simulink model "CM680A_HwTq2Meas"  (R2013b)
settings: Solver=FixedStepDiscrete  SolverMode=SingleTasking  StartTime=0.0  StopTime=1  FixedStep=0.002  RelTol=1e-3
values from neighbouring files (symbols this model uses):
  ELECGLBPRM_HWTQOFFS_HWNWTMTR_F32 = DataDict.Constant    [CM680A_HwTq2Meas_DataDict.m]
  ELECGLBPRM_HWTQSATNLOWRLIM_HWNWTMTR_F32 = DataDict.Constant    [CM680A_HwTq2Meas_DataDict.m]
  ELECGLBPRM_HWTQSATNUPPRLIM_HWNWTMTR_F32 = DataDict.Constant    [CM680A_HwTq2Meas_DataDict.m]
  ELECGLBPRM_HWTQSCA_ULS_F32 = DataDict.Constant    [CM680A_HwTq2Meas_DataDict.m]
  ELECGLBPRM_NOFLT_CNT_U08 = DataDict.Constant    [CM680A_HwTq2Meas_DataDict.m]
  ELECGLBPRM_OFFSTRIMNOTPRFM_CNT_U08 = DataDict.Constant    [CM680A_HwTq2Meas_DataDict.m]
  ELECGLBPRM_PRTCLFLT_CNT_U08 = DataDict.Constant    [CM680A_HwTq2Meas_DataDict.m]
  ELECGLBPRM_SNSRINTFLT_CNT_U08 = DataDict.Constant    [CM680A_HwTq2Meas_DataDict.m]
  FLTINJ_HWTQ2MEAS_HWTQ2 = DataDict.Constant    [CM680A_HwTq2Meas_DataDict.m]
  GearIdn1 = DataDict.OpSignal    [CM680A_HwTq2Meas_DataDict.m]
  HwTq2MeasHwTq2PrtclFltFailStep = DataDict.Calibration    [CM680A_HwTq2Meas_DataDict.m]
  HwTq2MeasHwTq2PrtclFltPassStep = DataDict.Calibration    [CM680A_HwTq2Meas_DataDict.m]
undefined symbols (not defined in the file or in its folder): NtcNr1, NtcSts1, sigbuilder_block, SigQlfr1
libraries: simulink x22, NxtrNvM x3
(part 2 of 3)

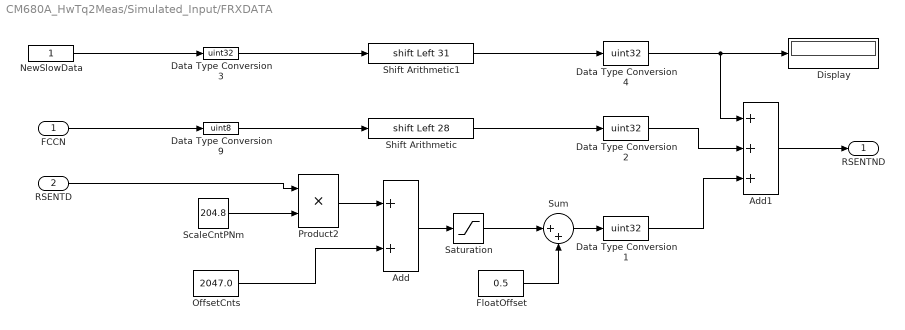
== system CM680A_HwTq2Meas/Simulated_Input/FRXDATA ==
  FCCN : Inport
  RSENTD : Inport  Port=2
  Add : Sum
  Add1 : Sum  Inputs=+++
  Data Type Conversion{1..4} (4 alike) : DataTypeConversion  OutDataTypeStr=uint32
  Data Type Conversion9 : DataTypeConversion  OutDataTypeStr=uint8
  Display : Display
  FloatOffset : Constant  Value=0.5
  NewSlowData : Constant
  OffsetCnts : Constant  Value=2047.0
  Product2 : Product
  Saturation : Saturate  UpperLimit=4095.0  LowerLimit=0.0
  ScaleCntPNm : Constant  Value=204.8
  Shift Arithmetic : ArithShift  BitShiftNumber=28  BitShiftDirection=Left
  Shift Arithmetic1 : ArithShift  BitShiftNumber=31  BitShiftDirection=Left
  Sum : Sum  Inputs=|++
  RSENTND : Outport
  wires:
  Data Type Conversion4/1 -> Add1/1, Display/1
  Shift Arithmetic1/1 -> Data Type Conversion4/1
  Data Type Conversion3/1 -> Shift Arithmetic1/1
  NewSlowData/1 -> Data Type Conversion3/1
  Data Type Conversion2/1 -> Add1/2
  Shift Arithmetic/1 -> Data Type Conversion2/1
  Add1/1 -> RSENTND/1
  Data Type Conversion1/1 -> Add1/3
  Data Type Conversion9/1 -> Shift Arithmetic/1
  FCCN/1 -> Data Type Conversion9/1
  Sum/1 -> Data Type Conversion1/1
  FloatOffset/1 -> Sum/2
  Saturation/1 -> Sum/1
  Add/1 -> Saturation/1
  OffsetCnts/1 -> Add/2
  Product2/1 -> Add/1
  ScaleCntPNm/1 -> Product2/2
  RSENTD/1 -> Product2/1

== system CM680A_HwTq2Meas/Simulated_Input/FRXDATA1 ==
  Snsr0CS : Inport
  Snsr0FRS : Inport  Port=2
  Add1 : Sum
  Data Type Conversion1 : DataTypeConversion  OutDataTypeStr=uint32
  Data Type Conversion9 : DataTypeConversion  OutDataTypeStr=uint32
  Shift Arithmetic2 : ArithShift  BitShiftNumber=1  BitShiftDirection=Left
  RSENTCS : Outport
  wires:
  Shift Arithmetic2/1 -> Add1/1
  Data Type Conversion9/1 -> Shift Arithmetic2/1
  Data Type Conversion1/1 -> Add1/2
  Snsr0FRS/1 -> Data Type Conversion1/1
  Add1/1 -> RSENTCS/1
  Snsr0CS/1 -> Data Type Conversion9/1

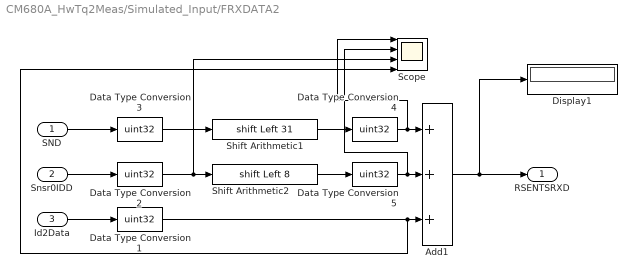
== system CM680A_HwTq2Meas/Simulated_Input/FRXDATA2 ==
  SND : Inport
  Snsr0IDD : Inport  Port=2
  Id2Data : Inport  Port=3
  Add1 : Sum  Inputs=+++
  Data Type Conversion{1..5} (5 alike) : DataTypeConversion  OutDataTypeStr=uint32
  Display1 : Display
  Scope : Scope  NumInputPorts=4
      settings: YMin=0~0~0~2  YMax=2.25e+09~1100~4~2
  Shift Arithmetic1 : ArithShift  BitShiftNumber=31  BitShiftDirection=Left
  Shift Arithmetic2 : ArithShift  BitShiftNumber=8  BitShiftDirection=Left
  RSENTSRXD : Outport
  wires:
  Id2Data/1 -> Data Type Conversion1/1
  Snsr0IDD/1 -> Data Type Conversion2/1
  Add1/1 -> RSENTSRXD/1, Display1/1
  SND/1 -> Data Type Conversion3/1
  Data Type Conversion3/1 -> Shift Arithmetic1/1
  Shift Arithmetic1/1 -> Data Type Conversion4/1
  Data Type Conversion4/1 -> Scope/1, Add1/1
  Data Type Conversion2/1 -> Scope/3, Shift Arithmetic2/1
  Data Type Conversion1/1 -> Scope/4, Add1/3
  Shift Arithmetic2/1 -> Data Type Conversion5/1
  Data Type Conversion5/1 -> Scope/2, Add1/2

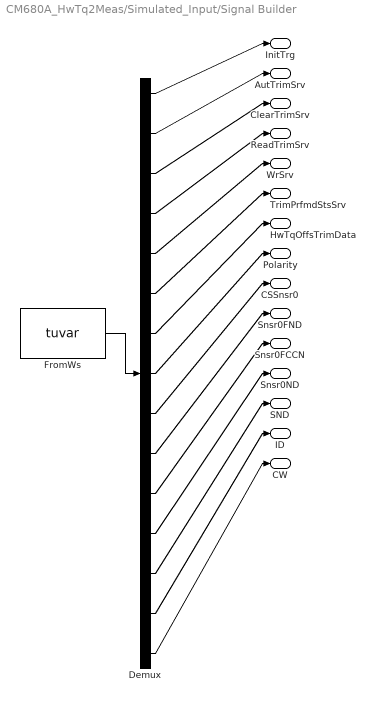
== system CM680A_HwTq2Meas/Simulated_Input/Signal Builder ==
  Demux : Demux  Tag=STV Demux  Outputs=15
  FromWs : FromWorkspace  Tag=STV FromWs  VariableName=tuvar  SampleTime=0  OutputAfterFinalValue=Holding final value
      SigBuilderData=|
      | common.afterFinalStr = 'Hold final value'
      | common.sampleTime = '0'
      | dataSet(1).timeRange = [0 20]
      | dataSet(1).name = 'IdealSignal'
      | dataSet(2).timeRange = [0 20]
      | dataSet(2).name = 'Faults'
      | dataSet(3).timeRange = [0 20]
      | dataSet(3).name = 'Service'
      | sbobj.Groups(1).Name = 'IdealSignal'
      | sbobj.Groups(1).Signals(1).Name = 'InitTrg'
      | sbobj.Groups(1).Signals(1).XData = [0 0.02 0.02 0.06 0.06 20]
      | sbobj.Groups(1).Signals(1).YData = [0 0 1 1 0 0]
      | sbobj.Groups(1).Signals(2).Name = 'AutTrimSrv'
      | sbobj.Groups(1).Signals(2).XData = [0 20]
      | sbobj.Groups(1).Signals(2).YData = [0 0]
      | sbobj.Groups(1).Signals(3).Name = 'ClearTrimSrv'
      | sbobj.Groups(1).Signals(3).XData = [0 20]
      | sbobj.Groups(1).Signals(3).YData = [0 0]
      | sbobj.Groups(1).Signals(4).Name = 'ReadTrimSrv'
      | sbobj.Groups(1).Signals(4).XData = [0 20]
      | sbobj.Groups(1).Signals(4).YData = [0 0]
      | sbobj.Groups(1).Signals(5).Name = 'WrSrv'
      | sbobj.Groups(1).Signals(5).XData = [0 0.04 0.04 0.08 0.08 20]
      | sbobj.Groups(1).Signals(5).YData = [0 0 1 1 0 0]
      | sbobj.Groups(1).Signals(6).Name = 'TrimPrfmdStsSrv'
      | sbobj.Groups(1).Signals(6).XData = [0 20]
      | sbobj.Groups(1).Signals(6).YData = [0 0]
      | sbobj.Groups(1).Signals(7).Name = 'HwTqOffsTrimData'
      | sbobj.Groups(1).Signals(7).XData = [0 20]
      | sbobj.Groups(1).Signals(7).YData = [0 0]
      | sbobj.Groups(1).Signals(8).Name = 'Polarity'
      | sbobj.Groups(1).Signals(8).XData = [0 20]
      | sbobj.Groups(1).Signals(8).YData = [1 1]
      | sbobj.Groups(1).Signals(9).Name = 'CSSnsr0'
      | sbobj.Groups(1).Signals(9).XData = [0 20]
      | sbobj.Groups(1).Signals(9).YData = [0 0]
      | sbobj.Groups(1).Signals(10).Name = 'Snsr0FND'
      | sbobj.Groups(1).Signals(10).XData = [0 20]
      | sbobj.Groups(1).Signals(10).YData = [1 1]
      | sbobj.Groups(1).Signals(11).Name = 'Snsr0FCCN'
      | sbobj.Groups(1).Signals(11).XData = [0 20]
      | sbobj.Groups(1).Signals(11).YData = [0 0]
      | sbobj.Groups(1).Signals(12).Name = 'Snsr0ND'
      | sbobj.Groups(1).Signals(12).XData = [0 2 2 4 4 6 6 8 8 10 10 12 12 14 14 16 16 18 18 20]
      | sbobj.Groups(1).Signals(12).YData = [-10 10 -10 10 -10 10 -10 10 -10 10 -10 10 -10 10 -10 10 -10 10 -10 10]
      | sbobj.Groups(1).Signals(13).Name = 'SND'
      | sbobj.Groups(1).Signals(13).XData = [0 0.1 0.1 0.2 0.2 0.3 0.3 0.4 0.4 0.5 0.5 0.6 0.6 0.7 0.7 0.8 0.8 0.9 0.9 1 1 1.1 1.1 1.2 1.2 1.3 1.3 1.4 1.4 1.5 1.5 1.6 1.6 1.7 1.7 1.8 1.8 1.9 1.9 2 2 2.1 2.1 2.2 2.2 2.3 2.3 2.4 2.4 2.5 2.5 2.6 2.6 2.7 2.7 2.8 2.8 2.9 2.9 3 3 3.1 3.1 3.2 3.2 3.3 3.3 3.4 3.4 3.5 3.5 3.6 3.6 3.7 3.7 3.8 3.8 3.9 3.9 4 4 4.1 4.1 4.2 4.2 4.3 4.3 4.4 4.4 4.5 4.5 4.6 4.6 4.7 4.7 4.8 4.8 4.9 4.9 5 5 5.1 5.1 5.2 5.2 5.3 5.3 5.4 5.4 5.5 5.5 5.6 5.6 5.7 5.7 5.8 5.8 5.9 5.9 6 6 6.1 6.1 6.2 6.2 6.3 6.3 6.4 6.4 6.5 6.5 6.6 6.6 6.7 6.7 6.8 6.8 6.9 6.9 7 7 7.1 7.1 7.2 7.2 7.3 7.3 7.4 7.4 7.5 7.5 7.6 7.6 7.7 7.7 7.8 7.8 7.9 7.9 8 8 8.1 8.1 8.2 8.2 8.3 8.3 8.4 8.4 8.5 8.5 8.6 8.6 8.7 8.7 8.8 8.8 8.9 8.9 9 9 9.1 9.1 9.2 9.2 9.3 9.3 9.4 9.4 9.5 9.5 9.6 9.6 9.7 9.7 9.8 9.8 9.9 9.9 10 10 10.1 10.1 10.2 10.2 10.3 10.3 10.4 10.4 10.5 10.5 10.6 10.6 10.7 10.7 10.8 10.8 10.9 10.9 11 11 11.1 11.1 11.2 11.2 11.3 11.3 11.4 11.4 11.5 11.5 11.6 11.6 11.7 11.7 11.8 11.8 11.9 11.9 12 12 12.1 12.1 12.2 12.2 12.3 12.3 12.4 12.4 12.5 12.5 12.6 12.6 12.7 12.7 12.8 12.8 12.9 12.9 13 13 13.1 13.1 13.2 13.2 13.3 13.3 13.4 13.4 13.5 13.5 13.6 13.6 13.7 13.7 13.8 13.8 13.9 13.9 14 14 14.1 14.1 14.2 14.2 14.3 14.3 14.4 14.4 14.5 14.5 14.6 14.6 14.7 14.7 14.8 14.8 14.9 14.9 15 15 15.1 15.1 15.2 15.2 15.3 15.3 15.4 15.4 15.5 15.5 15.6 15.6 15.7 15.7 15.8 15.8 15.9 15.9 16 16 16.1 16.1 16.2 16.2 16.3 16.3 16.4 16.4 16.5 16.5 16.6 16.6 16.7 16.7 16.8 16.8 16.9 16.9 17 17 17.1 17.1 17.2 17.2 17.3 17.3 17.4 17.4 17.5 17.5 17.6 17.6 17.7 17.7 17.8 17.8 17.9 17.9 18 18 18.1 18.1 18.2 18.2 18.3 18.3 18.4 18.4 18.5 18.5 18.6 18.6 18.7 18.7 18.8 18.8 18.9 18.9 19 19 19.1 19.1 19.2 19.2 19.3 19.3 19.4 19.4 19.5 19.5 19.6 19.6 19.7 19.7 19.8 19.8 19.9 19.9 20]
      | sbobj.Groups(1).Signals(13).YData = [1 1 0 0 1 1 0 0 1 1 0 0 1 1 0 0 1 1 0 0 1 1 0 0 1 1 0 0 1 1 0 0 1 1 0 0 1 1 0 0 1 1 0 0 1 1 0 0 1 1 0 0 1 1 0 0 1 1 0 0 1 1 0 0 1 1 0 0 1 1 0 0 1 1 0 0 1 1 0 0 1 1 0 0 1 1 0 0 1 1 0 0 1 1 0 0 1 1 0 0 1 1 0 0 1 1 0 0 1 1 0 0 1 1 0 0 1 1 0 0 1 1 0 0 1 1 0 0 1 1 0 0 1 1 0 0 1 1 0 0 1 1 0 0 1 1 0 0 1 1 0 0 1 1 0 0 1 1 0 0 1 1 0 0 1 1 0 0 1 1 0 0 1 1 0 0 1 1 0 0 1 1 0 0 1 1 0 0 1 1 0 0 1 1 0 0 1 1 0 0 1 1 0 0 1 1 0 0 1 1 0 0 1 1 0 0 1 1 0 0 1 1 0 0 1 1 0 0 1 1 0 0 1 1 0 0 1 1 0 0 1 1 0 0 1 1 0 0 1 1 0 0 1 1 0 0 1 1 0 0 1 1 0 0 1 1 0 0 1 1 0 0 1 1 0 0 1 1 0 0 1 1 0 0 1 1 0 0 1 1 0 0 1 1 0 0 1 1 0 0 1 1 0 0 1 1 0 0 1 1 0 0 1 1 0 0 1 1 0 0 1 1 0 0 1 1 0 0 1 1 0 0 1 1 0 0 1 1 0 0 1 1 0 0 1 1 0 0 1 1 0 0 1 1 0 0 1 1 0 0 1 1 0 0 1 1 0 0 1 1 0 0 1 1 0 0 1 1 0 0 1 1 0 0 1 1 0 0 1 1 0 0 1 1 0 0 1 1 0 0]
      | sbobj.Groups(1).Signals(14).Name = 'ID'
      | sbobj.Groups(1).Signals(14).XData = [0 0.166666666667 0.166666666667 0.333333333333 0.333333333333 0.5 0.5 0.666666666667 0.666666666667 0.833333333333 0.833333333333 1 ... (240 elements, 1x240)]
      | sbobj.Groups(1).Signals(14).YData = [1 1 0 0 1 1 0 0 3 3 0 0 2 2 0 0 4 4 0 0 1 1 0 0 1 1 0 0 1 1 0 0 1 1 0 0 1 1 0 0 1 1 0 0 1 1 0 0 1 1 0 0 1 1 0 0 1 1 0 0 1 1 0 0 1 1 0 0 1 1 0 0 1 1 0 0 1 1 0 0 1 1 0 0 1 1 0 0 1 1 0 0 1 1 0 0 1 1 0 0 1 1 0 0 1 1 0 0 1 1 0 0 1 1 0 0 1 1 0 0 1 1 0 0 1 1 0 0 2 2 0 0 3 3 0 0 4 4 0 0 1 1 0 0 1 1 0 0 1 1 0 0 1 1 0 0 1 1 0 0 1 1 0 0 1 1 0 0 1 1 0 0 1 1 0 0 1 1 0 0 1 1 0 0 1 1 0 0 1 1 0 0 1 1 0 0 1 1 0 0 1 1 0 0 1 1 0 0 1 1 0 0 1 1 0 0 1 1 0 0 1 1 0 0 1 1 0 0 1 1 0 0 1 1 0 0 1 1 0 0]
      | sbobj.Groups(1).Signals(15).Name = 'CW'
      | sbobj.Groups(1).Signals(15).XData = [0 5 5 10 10 15 15 20]
      | sbobj.Groups(1).Signals(15).YData = [2 2 0 0 4 4 6 6]
      | sbobj.Groups(1).TimeRange = [0 20]
      | sbobj.Groups(2).Name = 'Faults'
      | sbobj.Groups(2).Signals(1).Name = 'InitTrg'
      | sbobj.Groups(2).Signals(1).XData = [0 0.02 0.02 0.06 0.06 20]
      | sbobj.Groups(2).Signals(1).YData = [0 0 1 1 0 0]
      | sbobj.Groups(2).Signals(2).Name = 'AutTrimSrv'
      | sbobj.Groups(2).Signals(2).XData = [0 20]
      | sbobj.Groups(2).Signals(2).YData = [0 0]
      | sbobj.Groups(2).Signals(3).Name = 'ClearTrimSrv'
      | sbobj.Groups(2).Signals(3).XData = [0 20]
      | sbobj.Groups(2).Signals(3).YData = [0 0]
      | sbobj.Groups(2).Signals(4).Name = 'ReadTrimSrv'
      | sbobj.Groups(2).Signals(4).XData = [0 20]
      | sbobj.Groups(2).Signals(4).YData = [0 0]
      | sbobj.Groups(2).Signals(5).Name = 'WrSrv'
      | sbobj.Groups(2).Signals(5).XData = [0 0.06 0.06 0.12 0.12 20]
      | sbobj.Groups(2).Signals(5).YData = [0 0 1 1 0 0]
      | sbobj.Groups(2).Signals(6).Name = 'TrimPrfmdStsSrv'
      | sbobj.Groups(2).Signals(6).XData = [0 20]
      | sbobj.Groups(2).Signals(6).YData = [0 0]
      | sbobj.Groups(2).Signals(7).Name = 'HwTqOffsTrimData'
      | sbobj.Groups(2).Signals(7).XData = [0 20]
      | sbobj.Groups(2).Signals(7).YData = [0 0]
      | sbobj.Groups(2).Signals(8).Name = 'Polarity'
      | sbobj.Groups(2).Signals(8).XData = [0 11 11 20]
      | sbobj.Groups(2).Signals(8).YData = [-1 -1 1 1]
      | sbobj.Groups(2).Signals(9).Name = 'CSSnsr0'
      | sbobj.Groups(2).Signals(9).XData = [0 2.54 2.54 2.88 2.88 20]
      | sbobj.Groups(2).Signals(9).YData = [0 0 2 2 0 0]
      | sbobj.Groups(2).Signals(10).Name = 'Snsr0FND'
      | sbobj.Groups(2).Signals(10).XData = [0 14.54 14.54 14.78 14.78 20]
      | sbobj.Groups(2).Signals(10).YData = [1 1 0 0 1 1]
      | sbobj.Groups(2).Signals(11).Name = 'Snsr0FCCN'
      | sbobj.Groups(2).Signals(11).XData = [0 12.02 12.02 12.26 12.26 20]
      | sbobj.Groups(2).Signals(11).YData = [0 0 1 1 0 0]
      | sbobj.Groups(2).Signals(12).Name = 'Snsr0ND'
      | sbobj.Groups(2).Signals(12).XData = [0 2 2 4 4 6 6 8 8 10 10 12 12 14 14 16 16 18 18 20]
      | sbobj.Groups(2).Signals(12).YData = [-10 10 -10 10 -10 10 -10 10 -10 10 -10 10 -10 10 -10 10 -10 10 -10 10]
      | sbobj.Groups(2).Signals(13).Name = 'SND'
      | sbobj.Groups(2).Signals(13).XData = [0 0.1 0.1 0.2 0.2 0.3 0.3 0.4 0.4 0.5 0.5 0.6 0.6 0.7 0.7 0.8 0.8 0.9 0.9 1 1 1.1 1.1 1.2 1.2 1.3 1.3 1.4 1.4 1.5 1.5 1.6 1.6 1.7 1.7 1.8 1.8 1.9 1.9 2 2 2.1 2.1 2.2 2.2 2.3 2.3 2.4 2.4 2.5 2.5 2.6 2.6 2.7 2.7 2.8 2.8 2.9 2.9 3 3 3.1 3.1 3.2 3.2 3.3 3.3 3.4 3.4 3.5 3.5 3.6 3.6 3.7 3.7 3.8 3.8 3.9 3.9 4 4 4.1 4.1 4.2 4.2 4.3 4.3 4.4 4.4 4.5 4.5 4.6 4.6 4.7 4.7 4.8 4.8 4.9 4.9 5 5 5.1 5.1 5.2 5.2 5.3 5.3 5.4 5.4 5.5 5.5 5.6 5.6 5.7 5.7 5.8 5.8 5.9 5.9 6 6 6.1 6.1 6.2 6.2 6.3 6.3 6.4 6.4 6.5 6.5 6.6 6.6 6.7 6.7 6.8 6.8 6.9 6.9 7 7 7.1 7.1 7.2 7.2 7.3 7.3 7.4 7.4 7.5 7.5 7.6 7.6 7.7 7.7 7.8 7.8 7.9 7.9 8 8 8.1 8.1 8.2 8.2 8.3 8.3 8.4 8.4 8.5 8.5 8.6 8.6 8.7 8.7 8.8 8.8 8.9 8.9 9 9 9.1 9.1 9.2 9.2 9.3 9.3 9.4 9.4 9.5 9.5 9.6 9.6 9.7 9.7 9.8 9.8 9.9 9.9 10 10 10.1 10.1 10.2 10.2 10.3 10.3 10.4 10.4 10.5 10.5 10.6 10.6 10.7 10.7 10.8 10.8 10.9 10.9 11 11 11.1 11.1 11.2 11.2 11.3 11.3 11.4 11.4 11.5 11.5 11.6 11.6 11.7 11.7 11.8 11.8 11.9 11.9 12 12 12.1 12.1 12.2 12.2 12.3 12.3 12.4 12.4 12.5 12.5 12.6 12.6 12.7 12.7 12.8 12.8 12.9 12.9 13 13 13.1 13.1 13.2 13.2 13.3 13.3 13.4 13.4 13.5 13.5 13.6 13.6 13.7 13.7 13.8 13.8 13.9 13.9 14 14 14.1 14.1 14.2 14.2 14.3 14.3 14.4 14.4 14.5 14.5 14.6 14.6 14.7 14.7 14.8 14.8 14.9 14.9 15 15 15.1 15.1 15.2 15.2 15.3 15.3 15.4 15.4 15.5 15.5 15.6 15.6 15.7 15.7 15.8 15.8 15.9 15.9 16 16 16.1 16.1 16.2 16.2 16.3 16.3 16.4 16.4 16.5 16.5 16.6 16.6 16.7 16.7 16.8 16.8 16.9 16.9 17 17 17.1 17.1 17.2 17.2 17.3 17.3 17.4 17.4 17.5 17.5 17.6 17.6 17.7 17.7 17.8 17.8 17.9 17.9 18 18 18.1 18.1 18.2 18.2 18.3 18.3 18.4 18.4 18.5 18.5 18.6 18.6 18.7 18.7 18.8 18.8 18.9 18.9 19 19 19.1 19.1 19.2 19.2 19.3 19.3 19.4 19.4 19.5 19.5 19.6 19.6 19.7 19.7 19.8 19.8 19.9 19.9 20]
      | sbobj.Groups(2).Signals(13).YData = [1 1 0 0 1 1 0 0 1 1 0 0 1 1 0 0 1 1 0 0 1 1 0 0 1 1 0 0 1 1 0 0 1 1 0 0 1 1 0 0 1 1 0 0 1 1 0 0 1 1 0 0 1 1 0 0 1 1 0 0 1 1 0 0 1 1 0 0 1 1 0 0 1 1 0 0 1 1 0 0 1 1 0 0 1 1 0 0 1 1 0 0 1 1 0 0 1 1 0 0 1 1 0 0 1 1 0 0 1 1 0 0 1 1 0 0 1 1 0 0 1 1 0 0 1 1 0 0 1 1 0 0 1 1 0 0 1 1 0 0 1 1 0 0 1 1 0 0 1 1 0 0 1 1 0 0 1 1 0 0 1 1 0 0 1 1 0 0 1 1 0 0 1 1 0 0 1 1 0 0 1 1 0 0 1 1 0 0 1 1 0 0 1 1 0 0 1 1 0 0 1 1 0 0 1 1 0 0 1 1 0 0 1 1 0 0 1 1 0 0 1 1 0 0 1 1 0 0 1 1 0 0 1 1 0 0 1 1 0 0 1 1 0 0 1 1 0 0 1 1 0 0 1 1 0 0 1 1 0 0 1 1 0 0 1 1 0 0 1 1 0 0 1 1 0 0 1 1 0 0 1 1 0 0 1 1 0 0 1 1 0 0 1 1 0 0 1 1 0 0 1 1 0 0 1 1 0 0 1 1 0 0 1 1 0 0 1 1 0 0 1 1 0 0 1 1 0 0 1 1 0 0 1 1 0 0 1 1 0 0 1 1 0 0 1 1 0 0 1 1 0 0 1 1 0 0 1 1 0 0 1 1 0 0 1 1 0 0 1 1 0 0 1 1 0 0 1 1 0 0 1 1 0 0 1 1 0 0 1 1 0 0 1 1 0 0 1 1 0 0]
      | sbobj.Groups(2).Signals(14).Name = 'ID'
      | sbobj.Groups(2).Signals(14).XData = [0 0.166666666667 0.166666666667 0.333333333333 0.333333333333 0.5 0.5 0.666666666667 0.666666666667 0.833333333333 0.833333333333 1 ... (238 elements, 1x238)]
      | sbobj.Groups(2).Signals(14).YData = [1 1 0 0 1 1 0 0 3 3 0 0 2 2 0 0 0 0 1 1 0 0 1 1 0 0 1 1 0 0 1 1 0 0 1 1 0 0 1 1 0 0 1 1 0 0 1 1 0 0 1 1 0 0 1 1 0 0 1 1 0 0 1 1 0 0 1 1 0 0 1 1 0 0 1 1 0 0 1 1 0 0 1 1 0 0 1 1 0 0 1 1 0 0 1 1 0 0 1 1 0 0 1 1 0 0 1 1 0 0 1 1 0 0 1 1 0 0 1 1 0 0 1 1 0 0 1 1 0 0 1 1 0 0 1 1 0 0 1 1 0 0 1 1 0 0 1 1 0 0 1 1 0 0 1 1 0 0 1 1 0 0 1 1 0 0 1 1 0 0 1 1 0 0 1 1 0 0 1 1 0 0 1 1 0 0 1 1 0 0 1 1 0 0 1 1 0 0 1 1 0 0 1 1 0 0 1 1 0 0 1 1 0 0 1 1 0 0 1 1 0 0 1 1 0 0 1 1 0 0 1 1 0 0 1 1 0 0]
      | sbobj.Groups(2).Signals(15).Name = 'CW'
      | sbobj.Groups(2).Signals(15).XData = [0 5 5 10 10 15 15 20]
      | sbobj.Groups(2).Signals(15).YData = [2 2 0 0 4 4 6 6]
      | sbobj.Groups(2).TimeRange = [0 20]
      | sbobj.Groups(3).Name = 'Service'
      | sbobj.Groups(3).Signals(1).Name = 'InitTrg'
      | sbobj.Groups(3).Signals(1).XData = [0 0.02 0.02 0.06 0.06 20]
      | sbobj.Groups(3).Signals(1).YData = [0 0 1 1 0 0]
      | sbobj.Groups(3).Signals(2).Name = 'AutTrimSrv'
      | sbobj.Groups(3).Signals(2).XData = [0 0.58 0.58 0.68 0.68 16 16 16.1 16.1 20]
      | sbobj.Groups(3).Signals(2).YData = [0 0 1 1 0 0 1 1 0 0]
      | sbobj.Groups(3).Signals(3).Name = 'ClearTrimSrv'
      | sbobj.Groups(3).Signals(3).XData = [0 0.34 4.1 4.1 4.16 4.16 9.98 9.98 10.06 10.06 20]
      | sbobj.Groups(3).Signals(3).YData = [0 0 0 1 1 0 0 1 1 0 0]
      | sbobj.Groups(3).Signals(4).Name = 'ReadTrimSrv'
      | sbobj.Groups(3).Signals(4).XData = [0 1.24 1.24 1.32 1.32 4.62 4.62 4.7 4.7 6.84 6.84 6.92 6.92 10.38 10.38 10.46 10.46 16.72 16.72 16.8 16.8 20]
      | sbobj.Groups(3).Signals(4).YData = [0 0 1 1 0 0 1 1 0 0 1 1 0 0 1 1 0 0 1 1 0 0]
      | sbobj.Groups(3).Signals(5).Name = 'WrSrv'
      | sbobj.Groups(3).Signals(5).XData = [0 6.22 6.22 6.3 6.3 20]
      | sbobj.Groups(3).Signals(5).YData = [0 0 1 1 0 0]
      | sbobj.Groups(3).Signals(6).Name = 'TrimPrfmdStsSrv'
      | sbobj.Groups(3).Signals(6).XData = [0 1.24 1.24 1.32 1.32 4.64 4.64 4.7 4.7 6.84 6.84 6.92 6.92 10.64 10.64 10.72 10.72 16.74 16.74 16.82 16.82 20]
      | sbobj.Groups(3).Signals(6).YData = [0 0 1 1 0 0 1 1 0 0 1 1 0 0 1 1 0 0 1 1 0 0]
      | sbobj.Groups(3).Signals(7).Name = 'HwTqOffsTrimData'
      | sbobj.Groups(3).Signals(7).XData = [0 0.4 5.78 5.78 7.62 7.62 20]
      | sbobj.Groups(3).Signals(7).YData = [0 0 0 5 5 0 0]
      | sbobj.Groups(3).Signals(8).Name = 'Polarity'
      | sbobj.Groups(3).Signals(8).XData = [0 20]
      | sbobj.Groups(3).Signals(8).YData = [1 1]
      | sbobj.Groups(3).Signals(9).Name = 'CSSnsr0'
      | sbobj.Groups(3).Signals(9).XData = [0 20]
      | sbobj.Groups(3).Signals(9).YData = [0 0]
      | sbobj.Groups(3).Signals(10).Name = 'Snsr0FND'
      | sbobj.Groups(3).Signals(10).XData = [0 20]
      | sbobj.Groups(3).Signals(10).YData = [1 1]
      | sbobj.Groups(3).Signals(11).Name = 'Snsr0FCCN'
      | sbobj.Groups(3).Signals(11).XData = [0 20]
      | sbobj.Groups(3).Signals(11).YData = [0 0]
      | sbobj.Groups(3).Signals(12).Name = 'Snsr0ND'
      | sbobj.Groups(3).Signals(12).XData = [0 2 2 4 4 6 6 8 8 10 10 12 12 14 14 16 16 18 18 20]
      | sbobj.Groups(3).Signals(12).YData = [-10 10 -10 10 -10 10 -10 10 -10 10 -10 10 -10 10 -10 10 -10 10 -10 10]
      | sbobj.Groups(3).Signals(13).Name = 'SND'
      | sbobj.Groups(3).Signals(13).XData = [0 0.1 0.1 0.2 0.2 0.3 0.3 0.4 0.4 0.5 0.5 0.6 0.6 0.7 0.7 0.8 0.8 0.9 0.9 1 1 1.1 1.1 1.2 1.3 1.4 1.5 1.6 1.7 1.8 1.8 1.9 1.9 2 2 2.1 2.1 2.2 2.2 2.3 2.3 2.4 2.4 2.5 2.5 2.6 2.6 2.7 2.7 2.8 2.8 2.9 2.9 3 3 3.1 3.1 3.2 3.2 3.3 3.3 3.4 3.4 3.5 3.5 3.6 3.6 3.7 3.7 3.8 3.8 3.9 3.9 4 4 4.1 4.1 4.2 4.2 4.3 4.3 4.4 4.4 4.5 4.5 4.6 4.6 4.7 4.7 4.8 4.8 4.9 4.9 5 5 5.1 5.1 5.2 5.2 5.3 5.3 5.4 5.4 5.5 5.5 5.6 5.6 5.7 5.7 5.8 5.8 5.9 5.9 6 6 6.1 6.1 6.2 6.2 6.3 6.3 6.4 6.4 6.5 6.5 6.6 6.6 6.7 6.7 6.8 6.8 6.9 6.9 7 7 7.1 7.1 7.2 7.2 7.3 7.3 7.4 7.4 7.5 7.5 7.6 7.6 7.7 7.7 7.8 7.8 7.9 7.9 8 8 8.1 8.1 8.2 8.2 8.3 8.3 8.4 8.4 8.5 8.5 8.6 8.6 8.7 8.7 8.8 8.8 8.9 8.9 9 9 9.1 9.1 9.2 9.2 9.3 9.3 9.4 9.4 9.5 9.5 9.6 9.6 9.7 9.7 9.8 9.8 9.9 9.9 10 10 10.1 10.1 10.2 10.2 10.3 10.3 10.4 10.4 10.5 10.5 10.6 10.6 10.7 10.7 10.8 10.8 10.9 10.9 11 11 11.1 11.1 11.2 11.2 11.3 11.3 11.4 11.4 11.5 11.5 11.6 11.6 11.7 11.7 11.8 11.8 11.9 11.9 12 12 12.1 12.1 12.2 12.2 12.3 12.3 12.4 12.4 12.5 12.5 12.6 12.6 12.7 12.7 12.8 12.8 12.9 12.9 13 13 13.1 13.1 13.2 13.2 13.3 13.3 13.4 13.4 13.5 13.5 13.6 13.6 13.7 13.7 13.8 13.8 13.9 13.9 14 14 14.1 14.1 14.2 14.2 14.3 14.3 14.4 14.4 14.5 14.5 14.6 14.6 14.7 14.7 14.8 14.8 14.9 14.9 15 15 15.1 15.1 15.2 15.2 15.3 15.3 15.4 15.4 15.5 15.5 15.6 15.6 15.7 15.7 15.8 15.8 15.9 15.9 16 16 16.1 16.1 16.2 16.2 16.3 16.3 16.4 16.4 16.5 16.5 16.6 16.6 16.7 16.7 16.8 16.8 16.9 16.9 17 17 17.1 17.1 17.2 17.2 17.3 17.3 17.4 17.4 17.5 17.5 17.6 17.6 17.7 17.7 17.8 17.8 17.9 17.9 18 18 18.1 18.1 18.2 18.2 18.3 18.3 18.4 18.4 18.5 18.5 18.6 18.6 18.7 18.7 18.8 18.8 18.9 18.9 19 19 19.1 19.1 19.2 19.2 19.3 19.3 19.4 19.4 19.5 19.5 19.6 19.6 19.7 19.7 19.8 19.8 19.9 19.9 20]
      | sbobj.Groups(3).Signals(13).YData = [1 1 0 0 1 1 0 0 1 1 0 0 1 1 0 0 1 1 0 0 1 1 0 0 0 0 0 0 0 0 1 1 0 0 1 1 0 0 1 1 0 0 1 1 0 0 1 1 0 0 1 1 0 0 1 1 0 0 1 1 0 0 1 1 0 0 1 1 0 0 1 1 0 0 1 1 0 0 1 1 0 0 1 1 0 0 1 1 0 0 1 1 0 0 1 1 0 0 1 1 0 0 1 1 0 0 1 1 0 0 1 1 0 0 1 1 0 0 1 1 0 0 1 1 0 0 1 1 0 0 1 1 0 0 1 1 0 0 1 1 0 0 1 1 0 0 1 1 0 0 1 1 0 0 1 1 0 0 1 1 0 0 1 1 0 0 1 1 0 0 1 1 0 0 1 1 0 0 1 1 0 0 1 1 0 0 1 1 0 0 1 1 0 0 1 1 0 0 1 1 0 0 1 1 0 0 1 1 0 0 1 1 0 0 1 1 0 0 1 1 0 0 1 1 0 0 1 1 0 0 1 1 0 0 1 1 0 0 1 1 0 0 1 1 0 0 1 1 0 0 1 1 0 0 1 1 0 0 1 1 0 0 1 1 0 0 1 1 0 0 1 1 0 0 1 1 0 0 1 1 0 0 1 1 0 0 1 1 0 0 1 1 0 0 1 1 0 0 1 1 0 0 1 1 0 0 1 1 0 0 1 1 0 0 1 1 0 0 1 1 0 0 1 1 0 0 1 1 0 0 1 1 0 0 1 1 0 0 1 1 0 0 1 1 0 0 1 1 0 0 1 1 0 0 1 1 0 0 1 1 0 0 1 1 0 0 1 1 0 0 1 1 0 0 1 1 0 0 1 1 0 0 1 1 0 0 1 1 0 0 1 1 0 0]
      | sbobj.Groups(3).Signals(14).Name = 'ID'
      | sbobj.Groups(3).Signals(14).XData = [0 0.166666666667 0.166666666667 0.333333333333 0.333333333333 0.5 0.5 0.666666666667 0.666666666667 0.833333333333 0.833333333333 1 ... (240 elements, 1x240)]
      | sbobj.Groups(3).Signals(14).YData = [1 1 0 0 1 1 0 0 3 3 0 0 2 2 0 0 4 4 0 0 1 1 0 0 1 1 0 0 1 1 0 0 1 1 0 0 1 1 0 0 1 1 0 0 1 1 0 0 1 1 0 0 1 1 0 0 1 1 0 0 1 1 0 0 1 1 0 0 1 1 0 0 1 1 0 0 1 1 0 0 1 1 0 0 1 1 0 0 1 1 0 0 1 1 0 0 1 1 0 0 1 1 0 0 1 1 0 0 1 1 0 0 1 1 0 0 1 1 0 0 1 1 0 0 1 1 0 0 1 1 0 0 1 1 0 0 1 1 0 0 1 1 0 0 1 1 0 0 1 1 0 0 1 1 0 0 1 1 0 0 1 1 0 0 1 1 0 0 1 1 0 0 1 1 0 0 1 1 0 0 1 1 0 0 1 1 0 0 1 1 0 0 1 1 0 0 1 1 0 0 1 1 0 0 1 1 0 0 1 1 0 0 1 1 0 0 1 1 0 0 1 1 0 0 1 1 0 0 1 1 0 0 1 1 0 0 1 1 0 0]
      | sbobj.Groups(3).Signals(15).Name = 'CW'
      | sbobj.Groups(3).Signals(15).XData = [0 5 5 10 10 15 15 20]
      | sbobj.Groups(3).Signals(15).YData = [3 3 0 0 5 5 7 7]
      | sbobj.Groups(3).TimeRange = [0 20]
  InitTrg : Outport  Tag=STV Outport
  AutTrimSrv : Outport  Tag=STV Outport  Port=2
  ClearTrimSrv : Outport  Tag=STV Outport  Port=3
  ReadTrimSrv : Outport  Tag=STV Outport  Port=4
  WrSrv : Outport  Tag=STV Outport  Port=5
  TrimPrfmdStsSrv : Outport  Tag=STV Outport  Port=6
  HwTqOffsTrimData : Outport  Tag=STV Outport  Port=7
  Polarity : Outport  Tag=STV Outport  Port=8
  CSSnsr0 : Outport  Tag=STV Outport  Port=9
  Snsr0FND : Outport  Tag=STV Outport  Port=10
  Snsr0FCCN : Outport  Tag=STV Outport  Port=11
  Snsr0ND : Outport  Tag=STV Outport  Port=12
  SND : Outport  Tag=STV Outport  Port=13
  ID : Outport  Tag=STV Outport  Port=14
  CW : Outport  Tag=STV Outport  Port=15
  wires:
  Demux/15 -> CW/1
  Demux/14 -> ID/1
  Demux/13 -> SND/1
  Demux/12 -> Snsr0ND/1
  Demux/11 -> Snsr0FCCN/1
  Demux/10 -> Snsr0FND/1
  Demux/9 -> CSSnsr0/1
  Demux/8 -> Polarity/1
  Demux/7 -> HwTqOffsTrimData/1
  Demux/6 -> TrimPrfmdStsSrv/1
  Demux/5 -> WrSrv/1
  Demux/4 -> ReadTrimSrv/1
  Demux/3 -> ClearTrimSrv/1
  Demux/2 -> AutTrimSrv/1
  Demux/1 -> InitTrg/1
  FromWs/1 -> Demux/1

== system CM680A_HwTq2Meas/HwTq2Meas/HwTq2MeasHwTq2AutTrim/CopyRight2 ==

== system CM680A_HwTq2Meas/HwTq2Meas/HwTq2MeasHwTq2ClrTrim/CopyRight2 ==

== system CM680A_HwTq2Meas/HwTq2Meas/HwTq2MeasHwTq2ReadTrim/CopyRight2 ==

== system CM680A_HwTq2Meas/HwTq2Meas/HwTq2MeasHwTq2TrimPrfmdSts/CopyRight2 ==

== system CM680A_HwTq2Meas/HwTq2Meas/HwTq2MeasHwTq2WrTrim/CopyRight2 ==

== system CM680A_HwTq2Meas/HwTq2Meas/HwTq2MeasInit1/CopyRight2 ==

== system CM680A_HwTq2Meas/HwTq2Meas/HwTq2MeasInit1/GetRefTmr1MicroSec32bit ==
  CopyRight2 : Subsystem  Description=|  mask(Copyright Information){none=on}
      | Copyright info block.                                               
      |                                                                     
      | Place copyright information at the top of every subsystem in design.
      mask prompts: none "No parameters"
      mask help: Place copyright information at the top of every subsystem in design.
      mask Display:
      | NxtrConf = 'Nexteer Confidential';
      | 
      | sys = bdroot; %handle for the current model ("system")
      | first = get_param(sys,'Created');
      | first = first(end-3:end);  %year is last four digits
      | 
      | last = get_param(sys,'LastModifiedDate');
      | if isempty(last)
      |     last = datestr(now,'yyyy');
      | else
      |     last = last(end-3:end);
      | end
      | 
      | if strcmp(first,last)
      |     fprintf('%s -- Copyright %s Nexteer',NxtrConf,first)
      | else
      |     fprintf('%s -- %s%s- %s Nexteer',NxtrConf,char(169),first,last)
      | end
  Ground : Ground
  RefTmr : Outport
  wires:
  Ground/1 -> RefTmr/1

== system CM680A_HwTq2Meas/HwTq2Meas/HwTq2MeasInit1/GetTiSpan1MicroSec32bit ==
  RefTmr : Inport
  CopyRight2 : Subsystem  Description=|  mask(Copyright Information){none=on}
      | Copyright info block.                                               
      |                                                                     
      | Place copyright information at the top of every subsystem in design.
      mask prompts: none "No parameters"
      mask help: Place copyright information at the top of every subsystem in design.
      mask Display:
      | NxtrConf = 'Nexteer Confidential';
      | 
      | sys = bdroot; %handle for the current model ("system")
      | first = get_param(sys,'Created');
      | first = first(end-3:end);  %year is last four digits
      | 
      | last = get_param(sys,'LastModifiedDate');
      | if isempty(last)
      |     last = datestr(now,'yyyy');
      | else
      |     last = last(end-3:end);
      | end
      | 
      | if strcmp(first,last)
      |     fprintf('%s -- Copyright %s Nexteer',NxtrConf,first)
      | else
      |     fprintf('%s -- %s%s- %s Nexteer',NxtrConf,char(169),first,last)
      | end
  Ground : Ground
  Terminator : Terminator
  TiSpan : Outport
  wires:
  Ground/1 -> TiSpan/1
  RefTmr/1 -> Terminator/1

== system CM680A_HwTq2Meas/HwTq2Meas/HwTq2MeasInit1/IoHwAb_SetFctPrphlHwTq2 ==
  CopyRight2 : Subsystem  Description=|  mask(Copyright Information){none=on}
      | Copyright info block.                                               
      |                                                                     
      | Place copyright information at the top of every subsystem in design.
      mask prompts: none "No parameters"
      mask help: Place copyright information at the top of every subsystem in design.
      mask Display:
      | NxtrConf = 'Nexteer Confidential';
      | 
      | sys = bdroot; %handle for the current model ("system")
      | first = get_param(sys,'Created');
      | first = first(end-3:end);  %year is last four digits
      | 
      | last = get_param(sys,'LastModifiedDate');
      | if isempty(last)
      |     last = datestr(now,'yyyy');
      | else
      |     last = last(end-3:end);
      | end
      | 
      | if strcmp(first,last)
      |     fprintf('%s -- Copyright %s Nexteer',NxtrConf,first)
      | else
      |     fprintf('%s -- %s%s- %s Nexteer',NxtrConf,char(169),first,last)
      | end

== system CM680A_HwTq2Meas/HwTq2Meas/HwTq2MeasPer1/CopyRight2 ==

== system CM680A_HwTq2Meas/HwTq2Meas/HwTq2MeasPer1/DebStepSelection ==
  TestOk : Inport
  CopyRight2 : Subsystem  Description=|  mask(Copyright Information){none=on}
      | Copyright info block.                                               
      |                                                                     
      | Place copyright information at the top of every subsystem in design.
      mask prompts: none "No parameters"
      mask help: Place copyright information at the top of every subsystem in design.
      mask Display:
      | NxtrConf = 'Nexteer Confidential';
      | 
      | sys = bdroot; %handle for the current model ("system")
      | first = get_param(sys,'Created');
      | first = first(end-3:end);  %year is last four digits
      | 
      | last = get_param(sys,'LastModifiedDate');
      | if isempty(last)
      |     last = datestr(now,'yyyy');
      | else
      |     last = last(end-3:end);
      | end
      | 
      | if strcmp(first,last)
      |     fprintf('%s -- Copyright %s Nexteer',NxtrConf,first)
      | else
      |     fprintf('%s -- %s%s- %s Nexteer',NxtrConf,char(169),first,last)
      | end
  NTCFailStepCal : Constant  Value=HwTq2MeasHwTq2PrtclFltFailStep  VectorParams1D=off
  NTCPassStepCal : Constant  Value=HwTq2MeasHwTq2PrtclFltPassStep
  Switch : Switch  Criteria=u2 > Threshold  Threshold=2
  DebStep : Outport
  wires:
  TestOk/1 -> Switch/2
  NTCPassStepCal/1 -> Switch/3
  Switch/1 -> DebStep/1
  NTCFailStepCal/1 -> Switch/1

== system CM680A_HwTq2Meas/HwTq2Meas/HwTq2MeasPer1/Do nothing ==
  Action Port : ActionPort  ActionType=else
  CopyRight2 : Subsystem  Description=|  mask(Copyright Information){none=on}
      | Copyright info block.                                               
      |                                                                     
      | Place copyright information at the top of every subsystem in design.
      mask prompts: none "No parameters"
      mask help: Place copyright information at the top of every subsystem in design.
      mask Display:
      | NxtrConf = 'Nexteer Confidential';
      | 
      | sys = bdroot; %handle for the current model ("system")
      | first = get_param(sys,'Created');
      | first = first(end-3:end);  %year is last four digits
      | 
      | last = get_param(sys,'LastModifiedDate');
      | if isempty(last)
      |     last = datestr(now,'yyyy');
      | else
      |     last = last(end-3:end);
      | end
      | 
      | if strcmp(first,last)
      |     fprintf('%s -- Copyright %s Nexteer',NxtrConf,first)
      | else
      |     fprintf('%s -- %s%s- %s Nexteer',NxtrConf,char(169),first,last)
      | end

== system CM680A_HwTq2Meas/HwTq2Meas/HwTq2MeasPer1/FltInj_Sim1 ==
  note: Inport #2 must be constant
      | Const: FltInjectionLocType
  note: EA4.x Fault Injection
  note: This block requires no modification by FDD author.
      |
      | This block does not actually simulate any fault injection.  It is simply a pass-thru.
      |
      | The Const port (#2) simply terminates its signal, but we are trying to force the FDD author
      | to properly use the FltInjectionLocType enumeration in FDD model.
  Signal : Inport
  Const : Inport  Port=2
  Terminator : Terminator
  Out1 : Outport
  wires:
  Const/1 -> Terminator/1
  Signal/1 -> Out1/1

== system CM680A_HwTq2Meas/HwTq2Meas/HwTq2MeasPer1/GetNtcQlfr ==
  NtcNr : Inport
  CopyRight2 : Subsystem  Description=|  mask(Copyright Information){none=on}
      | Copyright info block.                                               
      |                                                                     
      | Place copyright information at the top of every subsystem in design.
      mask prompts: none "No parameters"
      mask help: Place copyright information at the top of every subsystem in design.
      mask Display:
      | NxtrConf = 'Nexteer Confidential';
      | 
      | sys = bdroot; %handle for the current model ("system")
      | first = get_param(sys,'Created');
      | first = first(end-3:end);  %year is last four digits
      | 
      | last = get_param(sys,'LastModifiedDate');
      | if isempty(last)
      |     last = datestr(now,'yyyy');
      | else
      |     last = last(end-3:end);
      | end
      | 
      | if strcmp(first,last)
      |     fprintf('%s -- Copyright %s Nexteer',NxtrConf,first)
      | else
      |     fprintf('%s -- %s%s- %s Nexteer',NxtrConf,char(169),first,last)
      | end
  Data Store Read : DataStoreRead  DataStoreName=Ntc0x077Qlfr
  Terminator : Terminator
  NtcQlfr : Outport
  wires:
  NtcNr/1 -> Terminator/1
  Data Store Read/1 -> NtcQlfr/1

== system CM680A_HwTq2Meas/HwTq2Meas/HwTq2MeasPer1/GetNtcQlfr1 ==
  NtcNr : Inport
  CopyRight2 : Subsystem  Description=|  mask(Copyright Information){none=on}
      | Copyright info block.                                               
      |                                                                     
      | Place copyright information at the top of every subsystem in design.
      mask prompts: none "No parameters"
      mask help: Place copyright information at the top of every subsystem in design.
      mask Display:
      | NxtrConf = 'Nexteer Confidential';
      | 
      | sys = bdroot; %handle for the current model ("system")
      | first = get_param(sys,'Created');
      | first = first(end-3:end);  %year is last four digits
      | 
      | last = get_param(sys,'LastModifiedDate');
      | if isempty(last)
      |     last = datestr(now,'yyyy');
      | else
      |     last = last(end-3:end);
      | end
      | 
      | if strcmp(first,last)
      |     fprintf('%s -- Copyright %s Nexteer',NxtrConf,first)
      | else
      |     fprintf('%s -- %s%s- %s Nexteer',NxtrConf,char(169),first,last)
      | end
  Data Store Read : DataStoreRead  DataStoreName=Ntc0x1E2Qlfr
  Terminator : Terminator
  NtcQlfr : Outport
  wires:
  NtcNr/1 -> Terminator/1
  Data Store Read/1 -> NtcQlfr/1

== system CM680A_HwTq2Meas/HwTq2Meas/HwTq2MeasPer1/HwTqCalculation ==
  RawHwTq : Inport
  CopyRight2 : Subsystem  Description=|  mask(Copyright Information){none=on}
      | Copyright info block.                                               
      |                                                                     
      | Place copyright information at the top of every subsystem in design.
      mask prompts: none "No parameters"
      mask help: Place copyright information at the top of every subsystem in design.
      mask Display:
      | NxtrConf = 'Nexteer Confidential';
      | 
      | sys = bdroot; %handle for the current model ("system")
      | first = get_param(sys,'Created');
      | first = first(end-3:end);  %year is last four digits
      | 
      | last = get_param(sys,'LastModifiedDate');
      | if isempty(last)
      |     last = datestr(now,'yyyy');
      | else
      |     last = last(end-3:end);
      | end
      | 
      | if strcmp(first,last)
      |     fprintf('%s -- Copyright %s Nexteer',NxtrConf,first)
      | else
      |     fprintf('%s -- %s%s- %s Nexteer',NxtrConf,char(169),first,last)
      | end
  Data Type Conversion : DataTypeConversion  OutDataTypeStr=single
  Data Type Conversion1 : DataTypeConversion  OutDataTypeStr=single
  HwTqOffs : Constant  Value=ELECGLBPRM_HWTQOFFS_HWNWTMTR_F32  OutDataTypeStr=single
  HwTqSca : Constant  Value=ELECGLBPRM_HWTQSCA_ULS_F32  OutDataTypeStr=single
  Product : Product
  Scope1 : Scope  NumInputPorts=2
      settings: YMin=-5~-5  YMax=5~5  SaveName=ScopeData2
  Substract : Sum  Inputs=+-
  HwTqData : Outport  OutDataTypeStr=single
  wires:
  HwTqSca/1 -> Product/2
  Product/1 -> Data Type Conversion1/1
  HwTqOffs/1 -> Substract/2
  Substract/1 -> Data Type Conversion/1
  RawHwTq/1 -> Product/1, Scope1/1
  Data Type Conversion1/1 -> Substract/1
  Data Type Conversion/1 -> Scope1/2, HwTqData/1

== system CM680A_HwTq2Meas/HwTq2Meas/HwTq2MeasPer1/If Action Subsystem1 ==
  Action Port : ActionPort  ActionType=then
  CopyRight2 : Subsystem  Description=|  mask(Copyright Information){none=on}
      | Copyright info block.                                               
      |                                                                     
      | Place copyright information at the top of every subsystem in design.
      mask prompts: none "No parameters"
      mask help: Place copyright information at the top of every subsystem in design.
      mask Display:
      | NxtrConf = 'Nexteer Confidential';
      | 
      | sys = bdroot; %handle for the current model ("system")
      | first = get_param(sys,'Created');
      | first = first(end-3:end);  %year is last four digits
      | 
      | last = get_param(sys,'LastModifiedDate');
      | if isempty(last)
      |     last = datestr(now,'yyyy');
      | else
      |     last = last(end-3:end);
      | end
      | 
      | if strcmp(first,last)
      |     fprintf('%s -- Copyright %s Nexteer',NxtrConf,first)
      | else
      |     fprintf('%s -- %s%s- %s Nexteer',NxtrConf,char(169),first,last)
      | end
  Data Type Conversion : DataTypeConversion  OutDataTypeStr=uint8
  SigQlfr : simulink/Sources/Enumerated Constant  OutDataTypeStr=Enum: SigQlfr1  Value=SigQlfr1.SIGQLFR_PASSD  SampleTime=inf
  Qlfr : Outport
  wires:
  SigQlfr/1 -> Data Type Conversion/1
  Data Type Conversion/1 -> Qlfr/1

== system CM680A_HwTq2Meas/HwTq2Meas/HwTq2MeasPer1/If Action Subsystem3 ==
  Action Port : ActionPort  ActionType=else
  CopyRight2 : Subsystem  Description=|  mask(Copyright Information){none=on}
      | Copyright info block.                                               
      |                                                                     
      | Place copyright information at the top of every subsystem in design.
      mask prompts: none "No parameters"
      mask help: Place copyright information at the top of every subsystem in design.
      mask Display:
      | NxtrConf = 'Nexteer Confidential';
      | 
      | sys = bdroot; %handle for the current model ("system")
      | first = get_param(sys,'Created');
      | first = first(end-3:end);  %year is last four digits
      | 
      | last = get_param(sys,'LastModifiedDate');
      | if isempty(last)
      |     last = datestr(now,'yyyy');
      | else
      |     last = last(end-3:end);
      | end
      | 
      | if strcmp(first,last)
      |     fprintf('%s -- Copyright %s Nexteer',NxtrConf,first)
      | else
      |     fprintf('%s -- %s%s- %s Nexteer',NxtrConf,char(169),first,last)
      | end
  Data Type Conversion : DataTypeConversion  OutDataTypeStr=uint8
  SigQlfr : simulink/Sources/Enumerated Constant  OutDataTypeStr=Enum: SigQlfr1  Value=SigQlfr1.SIGQLFR_FAILD  SampleTime=inf
  Qlfr : Outport
  wires:
  SigQlfr/1 -> Data Type Conversion/1
  Data Type Conversion/1 -> Qlfr/1

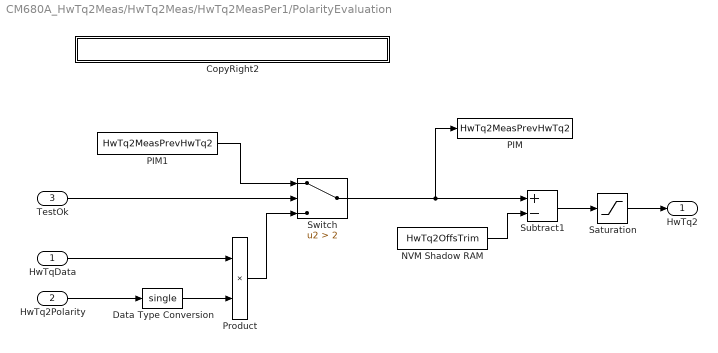
== system CM680A_HwTq2Meas/HwTq2Meas/HwTq2MeasPer1/PolarityEvaluation ==
  HwTqData : Inport  OutDataTypeStr=single
  HwTq2Polarity : Inport  RequirementInfo={} %GIDa_5e7beb6a_cd04_4438_bb0a_c4f4e2c14332  Port=2
  TestOk : Inport  Port=3
  CopyRight2 : Subsystem  Description=|  mask(Copyright Information){none=on}
      | Copyright info block.                                               
      |                                                                     
      | Place copyright information at the top of every subsystem in design.
      mask prompts: none "No parameters"
      mask help: Place copyright information at the top of every subsystem in design.
      mask Display:
      | NxtrConf = 'Nexteer Confidential';
      | 
      | sys = bdroot; %handle for the current model ("system")
      | first = get_param(sys,'Created');
      | first = first(end-3:end);  %year is last four digits
      | 
      | last = get_param(sys,'LastModifiedDate');
      | if isempty(last)
      |     last = datestr(now,'yyyy');
      | else
      |     last = last(end-3:end);
      | end
      | 
      | if strcmp(first,last)
      |     fprintf('%s -- Copyright %s Nexteer',NxtrConf,first)
      | else
      |     fprintf('%s -- %s%s- %s Nexteer',NxtrConf,char(169),first,last)
      | end
  Data Type Conversion : DataTypeConversion  OutDataTypeStr=single
  NVM Shadow RAM : DataStoreRead  DataStoreName=HwTq2OffsTrim
  PIM : DataStoreWrite  RequirementInfo={'linktype_rmi_doors' '0000cf42 (/ESG Group/FDD Module Requirements/EA4 Specific/CM680A_HwTq2Meas)' '#CM680A_52' 'true' 'REQ: CM680A_52' '' } %GIDa_077e43ec_662e_4d42_809b_03b059cade12  DataStoreName=HwTq2MeasPrevHwTq2
  PIM1 : DataStoreRead  DataStoreName=HwTq2MeasPrevHwTq2
  Product : Product  RequirementInfo={} %GIDa_582e6352_5967_4634_8e9a_a4093cfb2cb3
  Saturation : Saturate  UpperLimit=ELECGLBPRM_HWTQSATNUPPRLIM_HWNWTMTR_F32  LowerLimit=ELECGLBPRM_HWTQSATNLOWRLIM_HWNWTMTR_F32
  Subtract1 : Sum  Inputs=+-
  Switch : Switch  Criteria=u2 > Threshold  Threshold=2
  HwTq2 : Outport  RequirementInfo={'linktype_rmi_doors' '0000cf42 (/ESG Group/FDD Module Requirements/EA4 Specific/CM680A_HwTq2Meas)' '#CM680A_26' 'true' 'REQ: CM680A_26' '' } %GIDa_69c0e8a1_8bbe_4d59_a878_293d2bf0a501
  wires:
  Product/1 -> Switch/3
  TestOk/1 -> Switch/2
  Switch/1 -> PIM/1, Subtract1/1
  HwTq2Polarity/1 -> Data Type Conversion/1
  HwTqData/1 -> Product/1
  Data Type Conversion/1 -> Product/2
  Saturation/1 -> HwTq2/1
  Subtract1/1 -> Saturation/1
  NVM Shadow RAM/1 -> Subtract1/2
  PIM1/1 -> Switch/1

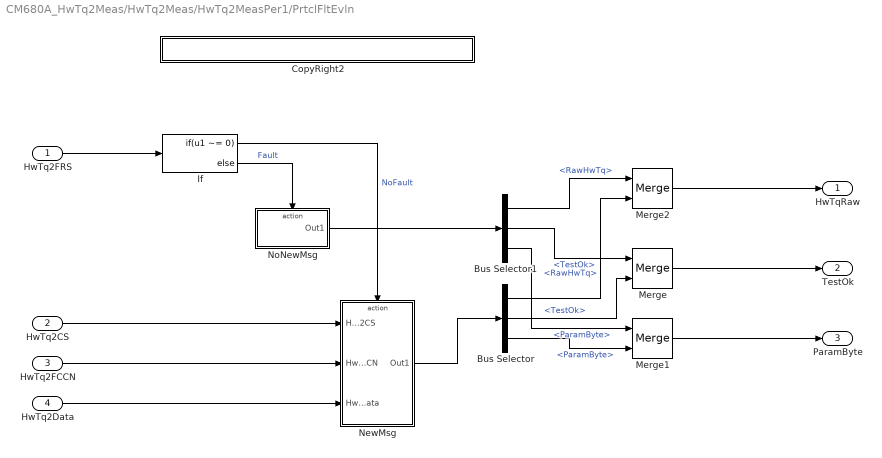
== system CM680A_HwTq2Meas/HwTq2Meas/HwTq2MeasPer1/PrtclFltEvln ==
  HwTq2FRS : Inport
  HwTq2CS : Inport  Port=2
  HwTq2FCCN : Inport  Port=3
  HwTq2Data : Inport  Port=4
  Bus Selector : BusSelector  OutputSignals=RawHwTq,TestOk,ParamByte
  Bus Selector1 : BusSelector  OutputSignals=RawHwTq,TestOk,ParamByte
  CopyRight2 : Subsystem  Description=|  mask(Copyright Information){none=on}
      | Copyright info block.                                               
      |                                                                     
      | Place copyright information at the top of every subsystem in design.
      mask prompts: none "No parameters"
      mask help: Place copyright information at the top of every subsystem in design.
      mask Display:
      | NxtrConf = 'Nexteer Confidential';
      | 
      | sys = bdroot; %handle for the current model ("system")
      | first = get_param(sys,'Created');
      | first = first(end-3:end);  %year is last four digits
      | 
      | last = get_param(sys,'LastModifiedDate');
      | if isempty(last)
      |     last = datestr(now,'yyyy');
      | else
      |     last = last(end-3:end);
      | end
      | 
      | if strcmp(first,last)
      |     fprintf('%s -- Copyright %s Nexteer',NxtrConf,first)
      | else
      |     fprintf('%s -- %s%s- %s Nexteer',NxtrConf,char(169),first,last)
      | end
  If : If  RequirementInfo={} %GIDa_27eddd86_3d73_4bbd_afc6_65cd0e917778  IfExpression=u1 ~= 0
  Merge : Merge
  Merge1 : Merge
  Merge2 : Merge
  NewMsg : Subsystem  RequirementInfo={'doors' '00006115' '17' 'false' 'DOORS Surrogate Item' '' } %GIDa_f428d820_7294_4433_be58_b2aad0418e6b  TreatAsAtomicUnit=on
      mask Display: disp('NewMsg')
  NoNewMsg : Subsystem  RequirementInfo={'linktype_rmi_doors' '0000cf42 (/ESG Group/FDD Module Requirements/EA4 Specific/CM680A_HwTq2Meas)' '#CM680A_47' 'true' 'REQ: CM680A_47' '' } %GIDa_9ee32e8d_1fd5_4b70_809d_63728be7576b  TreatAsAtomicUnit=on
      mask Display: disp('NoNewMsg')
  HwTqRaw : Outport
  TestOk : Outport  RequirementInfo={} %GIDa_95c6eb83_6b78_451b_a98a_b39fb65983b6  Port=2
  ParamByte : Outport  Port=3
  wires:
  HwTq2FRS/1 -> If/1
  If/1 -> NewMsg/Action  "NoFault"
  If/2 -> NoNewMsg/Action  "Fault"
  HwTq2CS/1 -> NewMsg/1(HwTq2CS)
  Merge/1 -> TestOk/1
  Merge1/1 -> ParamByte/1
  Merge2/1 -> HwTqRaw/1
  NewMsg/1(Out1) -> Bus Selector/1
  NoNewMsg/1(Out1) -> Bus Selector1/1
  Bus Selector1/1 -> Merge2/1  "<RawHwTq>"
  Bus Selector/1 -> Merge2/2  "<RawHwTq>"
  Bus Selector1/2 -> Merge/1  "<TestOk>"
  Bus Selector1/3 -> Merge1/1  "<ParamByte>"
  Bus Selector/2 -> Merge/2  "<TestOk>"
  Bus Selector/3 -> Merge1/2  "<ParamByte>"
  HwTq2FCCN/1 -> NewMsg/2(HwTq2FCCN)
  HwTq2Data/1 -> NewMsg/3(HwTq1Data)

== system CM680A_HwTq2Meas/HwTq2Meas/HwTq2MeasPer1/Read the Flag ==
  RegInpRSENT3FND : Inport
  Action Port : ActionPort  ActionType=then
  CopyRight2 : Subsystem  Description=|  mask(Copyright Information){none=on}
      | Copyright info block.                                               
      |                                                                     
      | Place copyright information at the top of every subsystem in design.
      mask prompts: none "No parameters"
      mask help: Place copyright information at the top of every subsystem in design.
      mask Display:
      | NxtrConf = 'Nexteer Confidential';
      | 
      | sys = bdroot; %handle for the current model ("system")
      | first = get_param(sys,'Created');
      | first = first(end-3:end);  %year is last four digits
      | 
      | last = get_param(sys,'LastModifiedDate');
      | if isempty(last)
      |     last = datestr(now,'yyyy');
      | else
      |     last = last(end-3:end);
      | end
      | 
      | if strcmp(first,last)
      |     fprintf('%s -- Copyright %s Nexteer',NxtrConf,first)
      | else
      |     fprintf('%s -- %s%s- %s Nexteer',NxtrConf,char(169),first,last)
      | end
  RSENT3DummyRead : Terminator
  wires:
  RegInpRSENT3FND/1 -> RSENT3DummyRead/1

== system CM680A_HwTq2Meas/HwTq2Meas/HwTq2MeasPer1/SetNtcSts ==
  note: Note:
      |
      | - "ISO Fault Debounce Design" Simulink block intent to use here for Simulation purpose only. Do not Code this block
  NtcNr : Inport
  NtcStInfo : Inport  Port=2
  NtcSts : Inport  Port=3
  DebStep : Inport  Port=4
  CopyRight2 : Subsystem  Description=|  mask(Copyright Information){none=on}
      | Copyright info block.                                               
      |                                                                     
      | Place copyright information at the top of every subsystem in design.
      mask prompts: none "No parameters"
      mask help: Place copyright information at the top of every subsystem in design.
      mask Display:
      | NxtrConf = 'Nexteer Confidential';
      | 
      | sys = bdroot; %handle for the current model ("system")
      | first = get_param(sys,'Created');
      | first = first(end-3:end);  %year is last four digits
      | 
      | last = get_param(sys,'LastModifiedDate');
      | if isempty(last)
      |     last = datestr(now,'yyyy');
      | else
      |     last = last(end-3:end);
      | end
      | 
      | if strcmp(first,last)
      |     fprintf('%s -- Copyright %s Nexteer',NxtrConf,first)
      | else
      |     fprintf('%s -- %s%s- %s Nexteer',NxtrConf,char(169),first,last)
      | end
  Data Store Write : DataStoreWrite  DataStoreName=Ntc0x077Qlfr
  Ground : Ground
  ISO Fault Debounce Design : Stateflow chart  TreatAsAtomicUnit=on
      settings: AttributesFormatString=|
      | Simulation Purpose Only.
      | Do Not Code this block
      | Diagnostic Manager Owns this requirement
  Scope1 : Scope  NumInputPorts=3
      settings: YMin=-5~-5~-5  YMax=5~5~5  SaveName=ScopeData5
  Terminator : Terminator
  Terminator1 : Terminator
  wires:
  NtcStInfo/1 -> Terminator1/1
  NtcNr/1 -> Terminator/1
  NtcSts/1 -> ISO Fault Debounce Design/1(NtcSts), Scope1/1
  DebStep/1 -> ISO Fault Debounce Design/2(DebStep), Scope1/2
  ISO Fault Debounce Design/1(Qualifier) -> Scope1/3, Data Store Write/1
  Ground/1 -> ISO Fault Debounce Design/3(SvcClr)

== system CM680A_HwTq2Meas/HwTq2Meas/HwTq2MeasPer1/SlowSerlDataRead ==
  note: Not Available
  note: False = Data is not available
      | True =  Data is available
  SlowSerlSND : Inport
  SlowSerlCS : Inport  Port=2
  SlowSerlMsgID : Inport  Port=3
  SlowSerlMsgData : Inport  Port=4
  CopyRight2 : Subsystem  Description=|  mask(Copyright Information){none=on}
      | Copyright info block.                                               
      |                                                                     
      | Place copyright information at the top of every subsystem in design.
      mask prompts: none "No parameters"
      mask help: Place copyright information at the top of every subsystem in design.
      mask Display:
      | NxtrConf = 'Nexteer Confidential';
      | 
      | sys = bdroot; %handle for the current model ("system")
      | first = get_param(sys,'Created');
      | first = first(end-3:end);  %year is last four digits
      | 
      | last = get_param(sys,'LastModifiedDate');
      | if isempty(last)
      |     last = datestr(now,'yyyy');
      | else
      |     last = last(end-3:end);
      | end
      | 
      | if strcmp(first,last)
      |     fprintf('%s -- Copyright %s Nexteer',NxtrConf,first)
      | else
      |     fprintf('%s -- %s%s- %s Nexteer',NxtrConf,char(169),first,last)
      | end
  If : If  RequirementInfo={} %GIDa_2422df38_1d15_44b2_a859_394211f873c4  IfExpression=~u1  ShowElse=off
  PIM : DataStoreRead  DataStoreName=GearIdn1Avl
  PIM1 : DataStoreRead  RequirementInfo={'linktype_rmi_doors' '0000cf42 (/ESG Group/FDD Module Requirements/EA4 Specific/CM680A_HwTq2Meas)' '#CM680A_68' 'true' 'REQ: CM680A_68' '' } %GIDa_6c48430c_4fec_4247_8593_9ebd888eb1e6  DataStoreName=GearIdn1Avl
  PIM2 : DataStoreRead  RequirementInfo={'linktype_rmi_doors' '0000cf42 (/ESG Group/FDD Module Requirements/EA4 Specific/CM680A_HwTq2Meas)' '#CM680A_68' 'true' 'REQ: CM680A_68' '' } %GIDa_57ab7112_e5f1_45ab_8099_a85e65dad929  DataStoreName=GearIdn1Data
  SlowSerlRead0 : Subsystem  RequirementInfo={} %GIDa_dd8e8880_4d93_4bc5_88e0_a17e4c8a2606  TreatAsAtomicUnit=on
  GearIdn1Vld : Outport  RequirementInfo={} %GIDa_9f99c856_3958_491c_a3f0_aceb6a3cf3b6
  GearIdn1 : Outport  RequirementInfo={} %GIDa_3749a270_a630_4e46_a559_cc9efc8df26c  Port=2
  wires:
  PIM2/1 -> GearIdn1/1  "GearIdn1"
  PIM1/1 -> GearIdn1Vld/1  "GearIdn1Vld"
  If/1 -> SlowSerlRead0/Action
  SlowSerlSND/1 -> SlowSerlRead0/1(SlowSerlSND)
  SlowSerlMsgID/1 -> SlowSerlRead0/3(SlowSerlMsgID)
  PIM/1 -> If/1
  SlowSerlCS/1 -> SlowSerlRead0/2(SlowSerlCS)
  SlowSerlMsgData/1 -> SlowSerlRead0/4(SlowSerlMsgData)

== system CM680A_HwTq2Meas/HwTq2Meas/HwTq2MeasPer2/CopyRight2 ==

== system CM680A_HwTq2Meas/HwTq2Meas/HwTq2MeasPer2/If Action Subsystem ==
  Action Port : ActionPort  ActionType=then
  CopyRight2 : Subsystem  Description=|  mask(Copyright Information){none=on}
      | Copyright info block.                                               
      |                                                                     
      | Place copyright information at the top of every subsystem in design.
      mask prompts: none "No parameters"
      mask help: Place copyright information at the top of every subsystem in design.
      mask Display:
      | NxtrConf = 'Nexteer Confidential';
      | 
      | sys = bdroot; %handle for the current model ("system")
      | first = get_param(sys,'Created');
      | first = first(end-3:end);  %year is last four digits
      | 
      | last = get_param(sys,'LastModifiedDate');
      | if isempty(last)
      |     last = datestr(now,'yyyy');
      | else
      |     last = last(end-3:end);
      | end
      | 
      | if strcmp(first,last)
      |     fprintf('%s -- Copyright %s Nexteer',NxtrConf,first)
      | else
      |     fprintf('%s -- %s%s- %s Nexteer',NxtrConf,char(169),first,last)
      | end
  Data Type Conversion : DataTypeConversion  OutDataTypeStr=uint8
  NoFlt : Constant  RequirementInfo={} %GIDa_73f0a11e_cf31_48e6_8bb2_3cf4b1949e36  Value=ELECGLBPRM_NOFLT_CNT_U08  OutDataTypeStr=uint8
  NtcSts : simulink/Sources/Enumerated Constant  OutDataTypeStr=Enum: NtcSts1  Value=NtcSts1.NTCSTS_PASSD  SampleTime=inf
  ParamByte : Outport
  TestOk : Outport  Port=2
  wires:
  NtcSts/1 -> Data Type Conversion/1
  NoFlt/1 -> ParamByte/1
  Data Type Conversion/1 -> TestOk/1

== system CM680A_HwTq2Meas/HwTq2Meas/HwTq2MeasPer2/If Action Subsystem1 ==
  Action Port : ActionPort  ActionType=else
  CopyRight2 : Subsystem  Description=|  mask(Copyright Information){none=on}
      | Copyright info block.                                               
      |                                                                     
      | Place copyright information at the top of every subsystem in design.
      mask prompts: none "No parameters"
      mask help: Place copyright information at the top of every subsystem in design.
      mask Display:
      | NxtrConf = 'Nexteer Confidential';
      | 
      | sys = bdroot; %handle for the current model ("system")
      | first = get_param(sys,'Created');
      | first = first(end-3:end);  %year is last four digits
      | 
      | last = get_param(sys,'LastModifiedDate');
      | if isempty(last)
      |     last = datestr(now,'yyyy');
      | else
      |     last = last(end-3:end);
      | end
      | 
      | if strcmp(first,last)
      |     fprintf('%s -- Copyright %s Nexteer',NxtrConf,first)
      | else
      |     fprintf('%s -- %s%s- %s Nexteer',NxtrConf,char(169),first,last)
      | end
  Data Type Conversion : DataTypeConversion  OutDataTypeStr=uint8
  NoFlt : Constant  RequirementInfo={} %GIDa_eae82ea4_69e1_4b6f_94ef_18d1f1394a46  Value=ELECGLBPRM_OFFSTRIMNOTPRFM_CNT_U08  OutDataTypeStr=uint8
  NtcSts : simulink/Sources/Enumerated Constant  OutDataTypeStr=Enum: NtcSts1  Value=NtcSts1.NTCSTS_FAILD  SampleTime=inf
  ParamByte : Outport
  TestOk : Outport  Port=2
  wires:
  NoFlt/1 -> ParamByte/1
  NtcSts/1 -> Data Type Conversion/1
  Data Type Conversion/1 -> TestOk/1

== system CM680A_HwTq2Meas/HwTq2Meas/HwTq2MeasPer2/SetNtcSts ==
  note: Note:
      |
      | - "ISO Fault Debounce Design" Simulink block intent to use here for Simulation purpose only. Do not Code this block
  NtcNr : Inport
  NtcStInfo : Inport  Port=2
  NtcSts : Inport  Port=3
  DebStep : Inport  Port=4
  CopyRight2 : Subsystem  Description=|  mask(Copyright Information){none=on}
      | Copyright info block.                                               
      |                                                                     
      | Place copyright information at the top of every subsystem in design.
      mask prompts: none "No parameters"
      mask help: Place copyright information at the top of every subsystem in design.
      mask Display:
      | NxtrConf = 'Nexteer Confidential';
      | 
      | sys = bdroot; %handle for the current model ("system")
      | first = get_param(sys,'Created');
      | first = first(end-3:end);  %year is last four digits
      | 
      | last = get_param(sys,'LastModifiedDate');
      | if isempty(last)
      |     last = datestr(now,'yyyy');
      | else
      |     last = last(end-3:end);
      | end
      | 
      | if strcmp(first,last)
      |     fprintf('%s -- Copyright %s Nexteer',NxtrConf,first)
      | else
      |     fprintf('%s -- %s%s- %s Nexteer',NxtrConf,char(169),first,last)
      | end
  Data Store Write : DataStoreWrite  DataStoreName=Ntc0x1E2Qlfr
  Ground : Ground
  ISO Fault Debounce Design : Stateflow chart  TreatAsAtomicUnit=on
      settings: AttributesFormatString=|
      | Simulation Purpose Only.
      | Do Not Code this block
      | Diagnostic Manager Owns this requirement
  Scope1 : Scope  NumInputPorts=3
      settings: YMin=-5~-5~-5  YMax=5~5~5  SaveName=ScopeData5
  Terminator : Terminator
  Terminator1 : Terminator
  wires:
  Ground/1 -> ISO Fault Debounce Design/3(SvcClr)
  ISO Fault Debounce Design/1(Qualifier) -> Data Store Write/1, Scope1/3
  DebStep/1 -> Scope1/2, ISO Fault Debounce Design/2(DebStep)
  NtcSts/1 -> Scope1/1, ISO Fault Debounce Design/1(NtcSts)
  NtcNr/1 -> Terminator/1
  NtcStInfo/1 -> Terminator1/1

== system CM680A_HwTq2Meas/HwTq2Meas/HwTq2MeasTrigStrt/CopyRight2 ==

== system CM680A_HwTq2Meas/HwTq2Meas/HwTq2MeasTrigStrt/GetRefTmr1MicroSec32bit ==
  CopyRight2 : Subsystem  Description=|  mask(Copyright Information){none=on}
      | Copyright info block.                                               
      |                                                                     
      | Place copyright information at the top of every subsystem in design.
      mask prompts: none "No parameters"
      mask help: Place copyright information at the top of every subsystem in design.
      mask Display:
      | NxtrConf = 'Nexteer Confidential';
      | 
      | sys = bdroot; %handle for the current model ("system")
      | first = get_param(sys,'Created');
      | first = first(end-3:end);  %year is last four digits
      | 
      | last = get_param(sys,'LastModifiedDate');
      | if isempty(last)
      |     last = datestr(now,'yyyy');
      | else
      |     last = last(end-3:end);
      | end
      | 
      | if strcmp(first,last)
      |     fprintf('%s -- Copyright %s Nexteer',NxtrConf,first)
      | else
      |     fprintf('%s -- %s%s- %s Nexteer',NxtrConf,char(169),first,last)
      | end
  Ground : Ground
  RefTmr : Outport
  wires:
  Ground/1 -> RefTmr/1

== system CM680A_HwTq2Meas/HwTq2Meas/HwTq2MeasTrigStrt/GetTiSpan1MicroSec32bit ==
  RefTmr : Inport
  CopyRight2 : Subsystem  Description=|  mask(Copyright Information){none=on}
      | Copyright info block.                                               
      |                                                                     
      | Place copyright information at the top of every subsystem in design.
      mask prompts: none "No parameters"
      mask help: Place copyright information at the top of every subsystem in design.
      mask Display:
      | NxtrConf = 'Nexteer Confidential';
      | 
      | sys = bdroot; %handle for the current model ("system")
      | first = get_param(sys,'Created');
      | first = first(end-3:end);  %year is last four digits
      | 
      | last = get_param(sys,'LastModifiedDate');
      | if isempty(last)
      |     last = datestr(now,'yyyy');
      | else
      |     last = last(end-3:end);
      | end
      | 
      | if strcmp(first,last)
      |     fprintf('%s -- Copyright %s Nexteer',NxtrConf,first)
      | else
      |     fprintf('%s -- %s%s- %s Nexteer',NxtrConf,char(169),first,last)
      | end
  Ground : Ground
  Terminator : Terminator
  TiSpan : Outport
  wires:
  RefTmr/1 -> Terminator/1
  Ground/1 -> TiSpan/1

== system CM680A_HwTq2Meas/HwTq2Meas/HwTq2MeasInit1/GetRefTmr1MicroSec32bit/CopyRight2 ==

== system CM680A_HwTq2Meas/HwTq2Meas/HwTq2MeasInit1/GetTiSpan1MicroSec32bit/CopyRight2 ==

== system CM680A_HwTq2Meas/HwTq2Meas/HwTq2MeasInit1/IoHwAb_SetFctPrphlHwTq2/CopyRight2 ==

== system CM680A_HwTq2Meas/HwTq2Meas/HwTq2MeasPer1/DebStepSelection/CopyRight2 ==

== system CM680A_HwTq2Meas/HwTq2Meas/HwTq2MeasPer1/Do nothing/CopyRight2 ==

== system CM680A_HwTq2Meas/HwTq2Meas/HwTq2MeasPer1/GetNtcQlfr/CopyRight2 ==

== system CM680A_HwTq2Meas/HwTq2Meas/HwTq2MeasPer1/GetNtcQlfr1/CopyRight2 ==

== system CM680A_HwTq2Meas/HwTq2Meas/HwTq2MeasPer1/HwTqCalculation/CopyRight2 ==

== system CM680A_HwTq2Meas/HwTq2Meas/HwTq2MeasPer1/If Action Subsystem1/CopyRight2 ==

== system CM680A_HwTq2Meas/HwTq2Meas/HwTq2MeasPer1/If Action Subsystem3/CopyRight2 ==

== system CM680A_HwTq2Meas/HwTq2Meas/HwTq2MeasPer1/PolarityEvaluation/CopyRight2 ==

== system CM680A_HwTq2Meas/HwTq2Meas/HwTq2MeasPer1/PrtclFltEvln/CopyRight2 ==

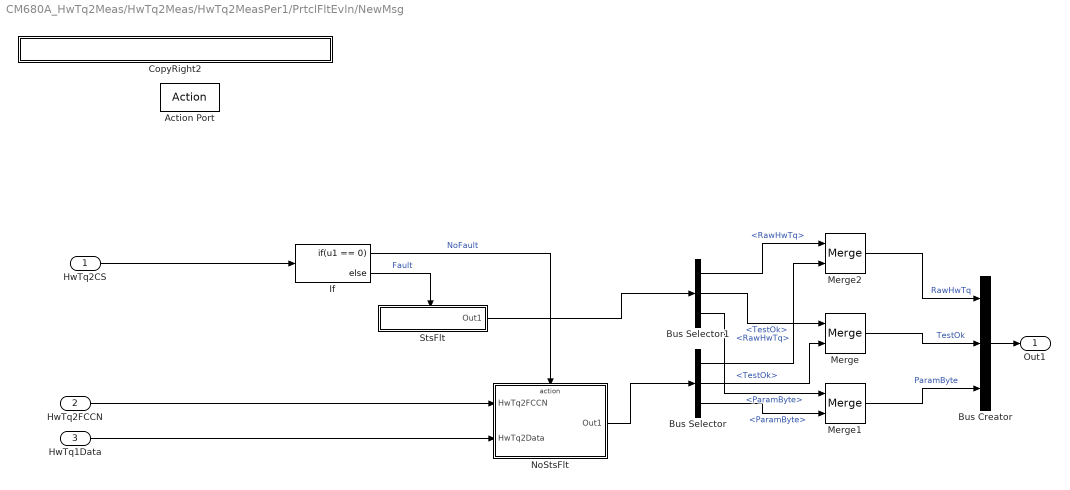
== system CM680A_HwTq2Meas/HwTq2Meas/HwTq2MeasPer1/PrtclFltEvln/NewMsg ==
  HwTq2CS : Inport
  HwTq2FCCN : Inport  Port=2
  HwTq1Data : Inport  Port=3
  Action Port : ActionPort  ActionType=then
  Bus Creator : BusCreator  Inputs=3
  Bus Selector : BusSelector  OutputSignals=RawHwTq,TestOk,ParamByte
  Bus Selector1 : BusSelector  OutputSignals=RawHwTq,TestOk,ParamByte
  CopyRight2 : Subsystem  Description=|  mask(Copyright Information){none=on}
      | Copyright info block.                                               
      |                                                                     
      | Place copyright information at the top of every subsystem in design.
      mask prompts: none "No parameters"
      mask help: Place copyright information at the top of every subsystem in design.
      mask Display:
      | NxtrConf = 'Nexteer Confidential';
      | 
      | sys = bdroot; %handle for the current model ("system")
      | first = get_param(sys,'Created');
      | first = first(end-3:end);  %year is last four digits
      | 
      | last = get_param(sys,'LastModifiedDate');
      | if isempty(last)
      |     last = datestr(now,'yyyy');
      | else
      |     last = last(end-3:end);
      | end
      | 
      | if strcmp(first,last)
      |     fprintf('%s -- Copyright %s Nexteer',NxtrConf,first)
      | else
      |     fprintf('%s -- %s%s- %s Nexteer',NxtrConf,char(169),first,last)
      | end
  If : If  IfExpression=u1 == 0
  Merge : Merge
  Merge1 : Merge
  Merge2 : Merge
  NoStsFlt : Subsystem  RequirementInfo={'doors' '00006115' '18' 'false' 'DOORS Surrogate Item' '' } %GIDa_ac6611b7_c860_4920_977e_a7e9bf2750f4  TreatAsAtomicUnit=on
  StsFlt : Subsystem  RequirementInfo={'linktype_rmi_doors' '0000cf42 (/ESG Group/FDD Module Requirements/EA4 Specific/CM680A_HwTq2Meas)' '#CM680A_40' 'true' 'REQ: CM680A_40' '' ; 'linktype_rmi_doors' '0000cf42 (/ESG Group/FDD Module Requirements/EA4 Specific/CM680A_HwTq2Meas)' '#CM680A_41' 'true' 'REQ: CM680A_41' '' ; 'linktype_rmi_doors' '0000cf42 (/ESG Group/FDD Module Requirements/EA4 Specific/CM680A_HwTq2Meas)' '#CM680A_42' 'true' 'REQ: CM680A_42' '' ; 'linktype_rmi_doors' '0000cf42 (/ESG Group/FDD Module Requirements/EA4 Specific/CM680A_HwTq2Meas)' '#CM680A_43' 'true' 'REQ: CM680A_43' '' ; 'linktype_rmi_doors' '0000cf42 (/ESG Group/FDD Module Requirements/EA4 Specific/CM680A_HwTq2Meas)' '#CM680A_44' 'true' 'REQ: CM680A_44' '' ; 'linktype_rmi_doors' '0000cf42 (/ESG Group/FDD Module Requirements/EA4 Specific/CM680A_HwTq2Meas)' '#CM680A_45' 'true' 'REQ: CM680A_45' '' ; 'linktype_rmi_doors' '0000cf42 (/ESG Group/FDD Module Requirements/EA4 Specific/CM680A_HwTq2Meas)' '#CM680A_46' 'true' 'REQ: CM680A_46' '' } %GIDa_679ffcb4_3849_4021_9957_65733ff452c6  TreatAsAtomicUnit=on
      mask Display: disp('STSFLT')
  Out1 : Outport
  wires:
  If/1 -> NoStsFlt/Action  "NoFault"
  If/2 -> StsFlt/Action  "Fault"
  Merge/1 -> Bus Creator/2  "TestOk"
  Merge1/1 -> Bus Creator/3  "ParamByte"
  Merge2/1 -> Bus Creator/1  "RawHwTq"
  NoStsFlt/1(Out1) -> Bus Selector/1
  StsFlt/1(Out1) -> Bus Selector1/1
  Bus Selector1/1 -> Merge2/1  "<RawHwTq>"
  Bus Selector/1 -> Merge2/2  "<RawHwTq>"
  Bus Selector1/2 -> Merge/1  "<TestOk>"
  Bus Selector1/3 -> Merge1/1  "<ParamByte>"
  Bus Selector/2 -> Merge/2  "<TestOk>"
  Bus Selector/3 -> Merge1/2  "<ParamByte>"
  Bus Creator/1 -> Out1/1
  HwTq2CS/1 -> If/1
  HwTq2FCCN/1 -> NoStsFlt/1(HwTq2FCCN)
  HwTq1Data/1 -> NoStsFlt/2(HwTq2Data)

== system CM680A_HwTq2Meas/HwTq2Meas/HwTq2MeasPer1/PrtclFltEvln/NoNewMsg ==
  Action Port : ActionPort  ActionType=else
  Add1 : Sum
  Bus Creator : BusCreator  Inputs=3
  Constant2 : Constant  OutDataTypeStr=uint32
  CopyRight2 : Subsystem  Description=|  mask(Copyright Information){none=on}
      | Copyright info block.                                               
      |                                                                     
      | Place copyright information at the top of every subsystem in design.
      mask prompts: none "No parameters"
      mask help: Place copyright information at the top of every subsystem in design.
      mask Display:
      | NxtrConf = 'Nexteer Confidential';
      | 
      | sys = bdroot; %handle for the current model ("system")
      | first = get_param(sys,'Created');
      | first = first(end-3:end);  %year is last four digits
      | 
      | last = get_param(sys,'LastModifiedDate');
      | if isempty(last)
      |     last = datestr(now,'yyyy');
      | else
      |     last = last(end-3:end);
      | end
      | 
      | if strcmp(first,last)
      |     fprintf('%s -- Copyright %s Nexteer',NxtrConf,first)
      | else
      |     fprintf('%s -- %s%s- %s Nexteer',NxtrConf,char(169),first,last)
      | end
  Data Type Conversion : DataTypeConversion  OutDataTypeStr=uint8
  NtcSts : simulink/Sources/Enumerated Constant  OutDataTypeStr=Enum: NtcSts1  Value=NtcSts1.NTCSTS_PREFAILD  SampleTime=inf
  PIM : DataStoreWrite  RequirementInfo={} %GIDa_b9149c9f_2c4e_401e_91f3_2794a0e512e2  DataStoreName=HwTq2MsgMissRxCnt
  PIM1 : DataStoreRead  DataStoreName=HwTq2MsgMissRxCnt
  PRTCL_FAULT : Constant  Value=ELECGLBPRM_PRTCLFLT_CNT_U08  OutDataTypeStr=uint8
  Signal Conversion : SignalConversion
  Trq : Constant  Value=0  OutDataTypeStr=uint32
  Out1 : Outport
  wires:
  NtcSts/1 -> Data Type Conversion/1
  PRTCL_FAULT/1 -> Bus Creator/3  "ParamByte"
  Data Type Conversion/1 -> Bus Creator/2  "TestOk"
  Trq/1 -> Bus Creator/1  "RawHwTq"
  Bus Creator/1 -> Signal Conversion/1
  Signal Conversion/1 -> Out1/1
  Add1/1 -> PIM/1
  Constant2/1 -> Add1/2
  PIM1/1 -> Add1/1

== system CM680A_HwTq2Meas/HwTq2Meas/HwTq2MeasPer1/Read the Flag/CopyRight2 ==

== system CM680A_HwTq2Meas/HwTq2Meas/HwTq2MeasPer1/SetNtcSts/CopyRight2 ==

== system CM680A_HwTq2Meas/HwTq2Meas/HwTq2MeasPer1/SlowSerlDataRead/CopyRight2 ==

== system CM680A_HwTq2Meas/HwTq2Meas/HwTq2MeasPer1/SlowSerlDataRead/SlowSerlRead0 ==
  SlowSerlSND : Inport
  SlowSerlCS : Inport  Port=2
  SlowSerlMsgID : Inport  Port=3
  SlowSerlMsgData : Inport  Port=4
  Action Port : ActionPort  ActionType=then
  CopyRight2 : Subsystem  Description=|  mask(Copyright Information){none=on}
      | Copyright info block.                                               
      |                                                                     
      | Place copyright information at the top of every subsystem in design.
      mask prompts: none "No parameters"
      mask help: Place copyright information at the top of every subsystem in design.
      mask Display:
      | NxtrConf = 'Nexteer Confidential';
      | 
      | sys = bdroot; %handle for the current model ("system")
      | first = get_param(sys,'Created');
      | first = first(end-3:end);  %year is last four digits
      | 
      | last = get_param(sys,'LastModifiedDate');
      | if isempty(last)
      |     last = datestr(now,'yyyy');
      | else
      |     last = last(end-3:end);
      | end
      | 
      | if strcmp(first,last)
      |     fprintf('%s -- Copyright %s Nexteer',NxtrConf,first)
      | else
      |     fprintf('%s -- %s%s- %s Nexteer',NxtrConf,char(169),first,last)
      | end
  If : If  NumInputs=2  IfExpression=(u1 ~= 0)&(u2==0)  ShowElse=off
      settings: AttributesFormatString=Condition: %<IfExpression>
  SlowSerlRead1 : Subsystem  RequirementInfo={} %GIDa_0e432c52_1423_451b_94c0_3a4098015282  TreatAsAtomicUnit=on
  wires:
  If/1 -> SlowSerlRead1/Action
  SlowSerlCS/1 -> If/2
  SlowSerlMsgID/1 -> SlowSerlRead1/1(SlowSerlMsgID)
  SlowSerlSND/1 -> If/1
  SlowSerlMsgData/1 -> SlowSerlRead1/2(SlowSerlMsgData)

== system CM680A_HwTq2Meas/HwTq2Meas/HwTq2MeasPer2/If Action Subsystem/CopyRight2 ==

== system CM680A_HwTq2Meas/HwTq2Meas/HwTq2MeasPer2/If Action Subsystem1/CopyRight2 ==

== system CM680A_HwTq2Meas/HwTq2Meas/HwTq2MeasPer2/SetNtcSts/CopyRight2 ==

== system CM680A_HwTq2Meas/HwTq2Meas/HwTq2MeasTrigStrt/GetRefTmr1MicroSec32bit/CopyRight2 ==

== system CM680A_HwTq2Meas/HwTq2Meas/HwTq2MeasTrigStrt/GetTiSpan1MicroSec32bit/CopyRight2 ==

== system CM680A_HwTq2Meas/HwTq2Meas/HwTq2MeasPer1/PrtclFltEvln/NewMsg/CopyRight2 ==
